simulink model "hug6dot_debug"  (R2021a)
settings: Solver=ode45  StartTime=0.0  StopTime=300  RelTol=1e-3
settings Model: Creator=daoist  LastModifiedBy=daoist

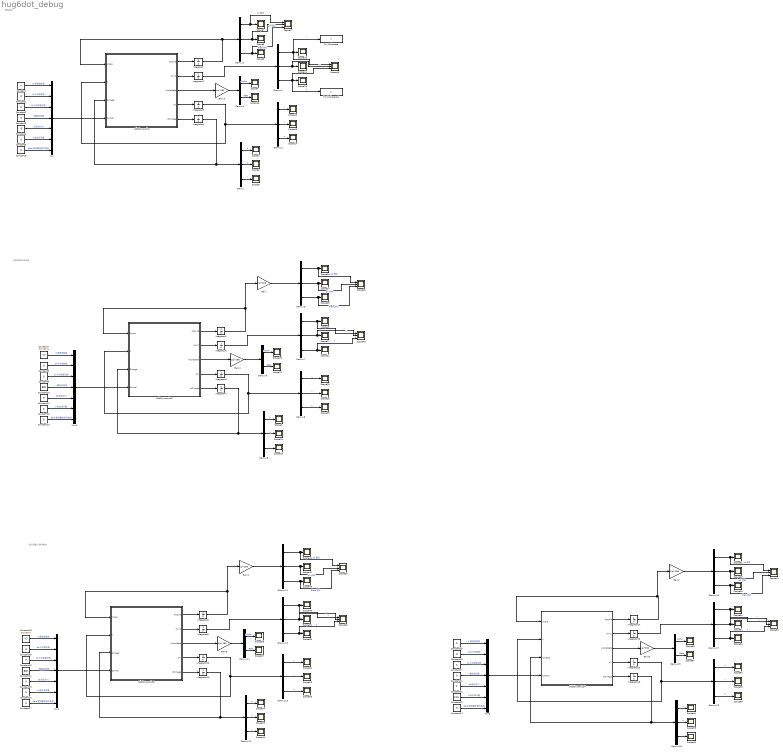
== system hug6dot_debug ==
  note: 验证忽略小项的影响
  note: 各种调试的实验场
  note: 原始版本
  6dotDynamics : Subsystem
  6dotDynamics2 : Subsystem
  6dotDynamics3 : Subsystem
  6dotDynamics4 : Subsystem
  Constant{,1..3,5..6,8..9,11..13,15..17,19..21,24..27} (21 alike) : Constant  Value=0
  Constant10 : Constant  Value=800
  Constant14 : Constant  Value=800
  Constant18 : Constant  Value=35/180*pi
  Constant22 : Constant  Value=2
  Constant23 : Constant  Value=0.01
  Constant4 : Constant  Value=-5
  Constant7 : Constant  Value=35/180*pi
  Demux{,1..3,5..8,10..13,15..18} (16 alike) : Demux  Outputs=3
  Demux{4,9,14,19} (4 alike) : Demux  Outputs=2
  Gain{,1..6} (7 alike) : Gain  Gain=1/pi*180
  Integrator{,1..2,4..5,7..9,11,13..15} (12 alike) : Integrator
  Integrator10 : Integrator  InitialCondition=[0.01 0 0]
  Integrator12 : Integrator  InitialCondition=[0.01 0 0]  UpperSaturationLimit=[inf 0.05 inf]  LowerSaturationLimit=-[inf 0.05 inf]
  Integrator3 : Integrator  InitialCondition=[0.01 0 0]
  Integrator6 : Integrator  InitialCondition=[0.01 0 0]
  Mux{,1..3} (4 alike) : Mux  Inputs=7
  Scope{1..28,31..43,45,51..64} (56 alike) : Scope
  Scope{29..30,44,46..50} (8 alike) : Scope  NumInputPorts=3
  To Workspace : ToWorkspace  VariableName=x  SampleTime=-1
  To Workspace1 : ToWorkspace  VariableName=z  SampleTime=-1
  wires:
  6dotDynamics/1(dAgnle) -> Integrator/1
  6dotDynamics/2(dXYZ) -> Integrator1/1
  6dotDynamics/4(dV) -> Integrator3/1
  6dotDynamics/5(dOmega) -> Integrator4/1
  Integrator4/1 -> 6dotDynamics/3(Omega), Demux/1
  Demux/1 -> Scope1/1  "p"
  Demux1/1 -> Scope47/1, Scope7/1  "psi横滚"
  Demux1/3 -> Scope47/3, Scope9/1  "theta俯仰"
  Integrator/1 -> Demux1/1, 6dotDynamics/1(Angle)
  Demux1/2 -> Scope47/2, Scope8/1  "phi回转"
  Demux3/1 -> Scope12/1  "u"
  Demux3/3 -> Scope14/1  "w"
  Integrator3/1 -> Demux3/1, 6dotDynamics/2(V)
  Demux3/2 -> Scope13/1  "v"
  Demux2/3 -> Scope46/3, To Workspace1/1, Scope15/1  "z"
  Demux2/1 -> Scope46/1, To Workspace/1, Scope10/1  "x"
  Demux2/2 -> Scope46/2, Scope11/1  "y"
  Integrator1/1 -> Demux2/1
  Demux/2 -> Scope5/1  "q"
  Demux/3 -> Scope6/1  "r"
  Demux4/1 -> Scope4/1  "Alpha"
  6dotDynamics/3(AlphaBeta) -> Gain3/1
  Demux4/2 -> Scope16/1  "Beta"
  Constant/1 -> Mux/1  "dr垂直舵舵角"
  Constant1/1 -> Mux/2  "de水平舵舵角"
  Constant2/1 -> Mux/3  "dd水平舵差动角"
  Constant3/1 -> Mux/4  "n螺旋桨转速"
  Constant4/1 -> Mux/5  "dB驱动浮力"
  Constant5/1 -> Mux/6  "dl姿态调节量"
  Constant6/1 -> Mux/7  "delta横滚重物调节角度"
  Mux/1 -> 6dotDynamics/4(Control)
  Mux1/1 -> 6dotDynamics2/4(Control)
  Constant13/1 -> Mux1/7  "delta横滚重物调节角度"
  Constant12/1 -> Mux1/6  "dl姿态调节量"
  Constant7/1 -> Mux1/1  "dr垂直舵舵角"
  Demux5/3 -> Scope25/1  "r"
  Demux5/2 -> Scope24/1  "q"
  Demux7/1 -> Scope49/1, Scope3/1  "x"
  6dotDynamics2/3(AlphaBeta) -> Gain4/1
  6dotDynamics2/5(dOmega) -> Integrator7/1
  Constant10/1 -> Mux1/4  "n螺旋桨转速"
  Demux7/2 -> Scope49/2, Scope17/1  "y"
  Demux9/1 -> Scope23/1  "Alpha"
  Demux7/3 -> Scope49/3, Scope21/1  "z"
  Demux9/2 -> Scope22/1  "Beta"
  Demux8/2 -> Scope19/1  "v"
  Demux6/1 -> Scope48/1, Scope26/1  "psi横滚"
  Demux6/3 -> Scope48/3, Scope28/1  "theta俯仰"
  Demux8/1 -> Scope18/1  "u"
  6dotDynamics2/1(dAgnle) -> Integrator2/1
  Demux5/1 -> Scope2/1  "p"
  Constant11/1 -> Mux1/5  "dB驱动浮力"
  Demux8/3 -> Scope20/1  "w"
  6dotDynamics2/4(dV) -> Integrator6/1
  Demux6/2 -> Scope48/2, Scope27/1  "phi回转"
  Integrator7/1 -> 6dotDynamics2/3(Omega), Demux5/1
  Constant9/1 -> Mux1/3  "dd水平舵差动角"
  Constant8/1 -> Mux1/2  "de水平舵舵角"
  Integrator6/1 -> Demux8/1, 6dotDynamics2/2(V)
  Integrator5/1 -> Demux7/1
  Integrator2/1 -> Gain/1, 6dotDynamics2/1(Angle)
  6dotDynamics2/2(dXYZ) -> Integrator5/1
  Gain/1 -> Demux6/1
  Constant16/1 -> Mux2/6  "dl姿态调节量"
  Constant19/1 -> Mux2/2  "de水平舵舵角"
  Constant20/1 -> Mux2/3  "dd水平舵差动角"
  Demux13/1 -> Scope32/1  "u"
  Integrator11/1 -> 6dotDynamics3/3(Omega), Demux10/1
  Demux11/2 -> Scope29/2, Scope42/1  "phi回转"
  6dotDynamics3/1(dAgnle) -> Integrator8/1
  Constant15/1 -> Mux2/5  "dB驱动浮力"
  Demux11/3 -> Scope29/3, Scope43/1  "theta俯仰"
  Demux10/2 -> Scope39/1  "q"
  Demux13/3 -> Scope35/1  "w"
  Integrator8/1 -> Gain1/1, 6dotDynamics3/1(Angle)
  Demux12/2 -> Scope30/2, Scope31/1  "y"
  Constant18/1 -> Mux2/1  "dr垂直舵舵角"
  Demux13/2 -> Scope33/1  "v"
  Mux2/1 -> 6dotDynamics3/4(Control)
  Integrator9/1 -> Demux12/1
  Demux14/1 -> Scope38/1  "Alpha"
  Integrator10/1 -> Demux13/1, 6dotDynamics3/2(V)
  Demux10/1 -> Scope34/1  "p"
  6dotDynamics3/3(AlphaBeta) -> Gain5/1
  Demux12/3 -> Scope30/3, Scope36/1  "z"
  Demux11/1 -> Scope29/1, Scope41/1  "psi横滚"
  6dotDynamics3/4(dV) -> Integrator10/1
  Demux12/1 -> Scope30/1, Scope45/1  "x"
  Demux14/2 -> Scope37/1  "Beta"
  Constant14/1 -> Mux2/4  "n螺旋桨转速"
  6dotDynamics3/2(dXYZ) -> Integrator9/1
  Gain1/1 -> Demux11/1
  Demux10/3 -> Scope40/1  "r"
  Constant17/1 -> Mux2/7  "delta横滚重物调节角度"
  6dotDynamics3/5(dOmega) -> Integrator11/1
  6dotDynamics4/5(dOmega) -> Integrator13/1
  Demux17/2 -> Scope50/2, Scope51/1  "y"
  Demux19/2 -> Scope57/1  "Beta"
  Mux3/1 -> 6dotDynamics4/4(Control)
  Gain2/1 -> Demux16/1
  Constant24/1 -> Mux3/7  "delta横滚重物调节角度"
  Integrator13/1 -> 6dotDynamics4/3(Omega), Demux15/1
  6dotDynamics4/3(AlphaBeta) -> Gain6/1
  Demux18/2 -> Scope53/1  "v"
  Demux17/1 -> Scope50/1, Scope64/1  "x"
  Demux15/2 -> Scope59/1  "q"
  Constant21/1 -> Mux3/4  "n螺旋桨转速"
  Integrator15/1 -> Demux17/1
  6dotDynamics4/2(dXYZ) -> Integrator15/1
  Demux19/1 -> Scope58/1  "Alpha"
  Demux15/3 -> Scope60/1  "r"
  Integrator14/1 -> Gain2/1, 6dotDynamics4/1(Angle)
  Constant26/1 -> Mux3/2  "de水平舵舵角"
  Constant25/1 -> Mux3/1  "dr垂直舵舵角"
  6dotDynamics4/4(dV) -> Integrator12/1
  Demux15/1 -> Scope54/1  "p"
  Demux16/1 -> Scope44/1, Scope61/1  "psi横滚"
  Integrator12/1 -> Demux18/1, 6dotDynamics4/2(V)
  Constant23/1 -> Mux3/6  "dl姿态调节量"
  6dotDynamics4/1(dAgnle) -> Integrator14/1
  Constant27/1 -> Mux3/3  "dd水平舵差动角"
  Demux18/1 -> Scope52/1  "u"
  Demux18/3 -> Scope55/1  "w"
  Demux16/3 -> Scope44/3, Scope63/1  "theta俯仰"
  Demux17/3 -> Scope50/3, Scope56/1  "z"
  Constant22/1 -> Mux3/5  "dB驱动浮力"
  Demux16/2 -> Scope44/2, Scope62/1  "phi回转"
  Gain3/1 -> Demux4/1
  Gain4/1 -> Demux9/1
  Gain5/1 -> Demux14/1
  Gain6/1 -> Demux19/1

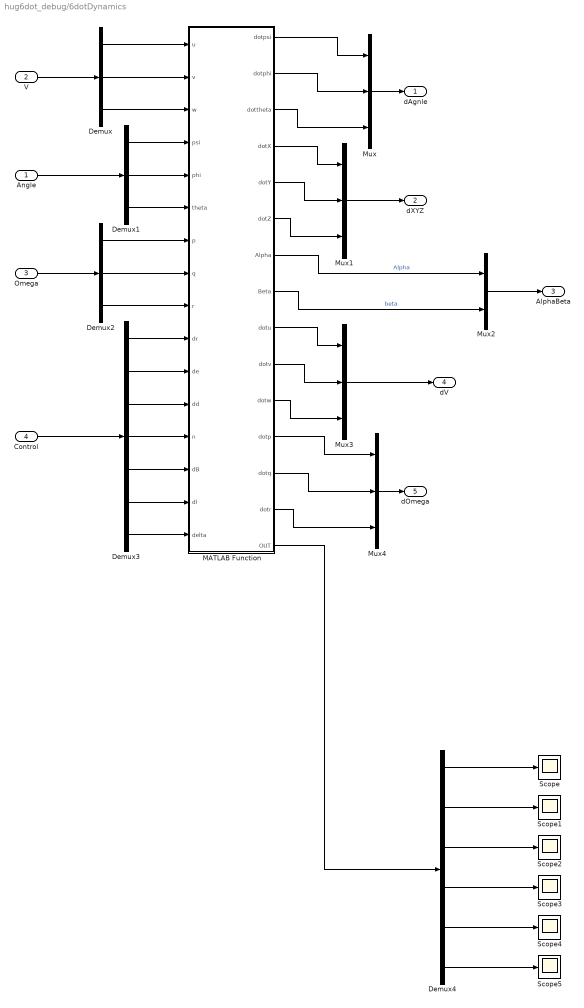
== system hug6dot_debug/6dotDynamics ==
  Angle : Inport
  V : Inport  Port=2
  Omega : Inport  Port=3
  Control : Inport  Port=4
  Demux : Demux  Outputs=3
  Demux1 : Demux  Outputs=3
  Demux2 : Demux  Outputs=3
  Demux3 : Demux  Outputs=7
  Demux4 : Demux  Outputs=6
  MATLAB Function : MATLAB Function  TreatAsAtomicUnit=on
  Mux{,1,3..4} (4 alike) : Mux  Inputs=3
  Mux2 : Mux  Inputs=2
  Scope{,1..5} (6 alike) : Scope
  dAgnle : Outport
  dXYZ : Outport  Port=2
  AlphaBeta : Outport  Port=3
  dV : Outport  Port=4
  dOmega : Outport  Port=5
  wires:
  MATLAB Function/6(dotZ) -> Mux1/3
  Mux1/1 -> dXYZ/1
  MATLAB Function/4(dotX) -> Mux1/1
  MATLAB Function/5(dotY) -> Mux1/2
  Mux/1 -> dAgnle/1
  MATLAB Function/7(Alpha) -> Mux2/1  "Alpha"
  MATLAB Function/8(Beta) -> Mux2/2  "beta"
  Mux2/1 -> AlphaBeta/1
  MATLAB Function/9(dotu) -> Mux3/1
  MATLAB Function/10(dotv) -> Mux3/2
  MATLAB Function/11(dotw) -> Mux3/3
  Mux3/1 -> dV/1
  MATLAB Function/12(dotp) -> Mux4/1
  MATLAB Function/13(dotq) -> Mux4/2
  MATLAB Function/14(dotr) -> Mux4/3
  Mux4/1 -> dOmega/1
  Demux/1 -> MATLAB Function/1(u)
  Demux/2 -> MATLAB Function/2(v)
  Demux/3 -> MATLAB Function/3(w)
  V/1 -> Demux/1
  Angle/1 -> Demux1/1
  Demux2/1 -> MATLAB Function/7(p)
  Demux2/2 -> MATLAB Function/8(q)
  Demux2/3 -> MATLAB Function/9(r)
  Omega/1 -> Demux2/1
  MATLAB Function/1(dotpsi) -> Mux/1
  MATLAB Function/2(dotphi) -> Mux/2
  MATLAB Function/3(dottheta) -> Mux/3
  Demux1/1 -> MATLAB Function/4(psi)
  Demux1/3 -> MATLAB Function/6(theta)
  Demux1/2 -> MATLAB Function/5(phi)
  Control/1 -> Demux3/1
  Demux3/1 -> MATLAB Function/10(dr)
  Demux3/2 -> MATLAB Function/11(de)
  Demux3/3 -> MATLAB Function/12(dd)
  Demux3/4 -> MATLAB Function/13(n)
  Demux3/5 -> MATLAB Function/14(dB)
  Demux3/6 -> MATLAB Function/15(dl)
  Demux3/7 -> MATLAB Function/16(delta)
  Demux4/1 -> Scope/1
  Demux4/5 -> Scope4/1
  Demux4/6 -> Scope5/1
  Demux4/4 -> Scope3/1
  Demux4/3 -> Scope2/1
  Demux4/2 -> Scope1/1
  MATLAB Function/15(OUT) -> Demux4/1

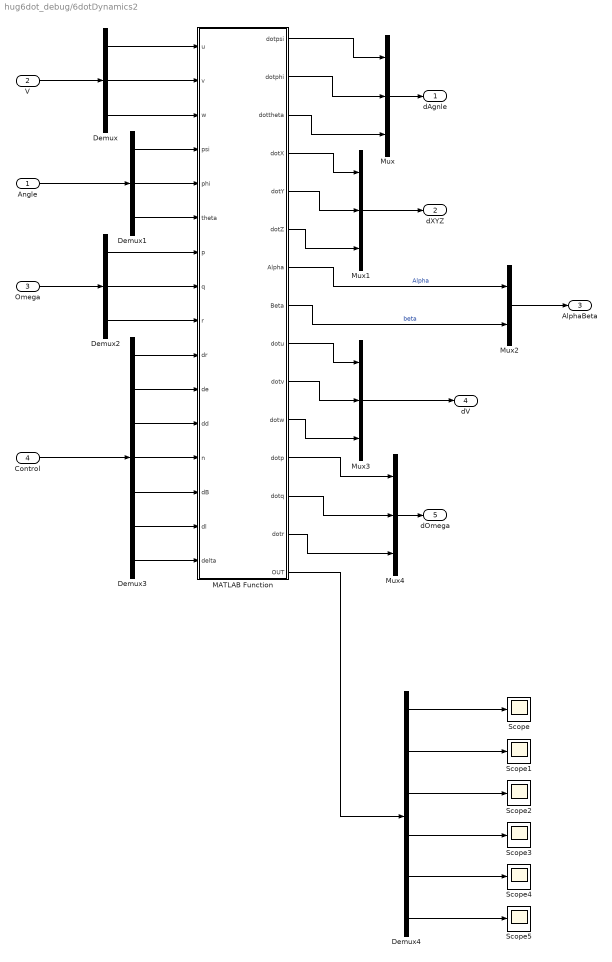
== system hug6dot_debug/6dotDynamics2 ==
  Angle : Inport
  V : Inport  Port=2
  Omega : Inport  Port=3
  Control : Inport  Port=4
  Demux : Demux  Outputs=3
  Demux1 : Demux  Outputs=3
  Demux2 : Demux  Outputs=3
  Demux3 : Demux  Outputs=7
  Demux4 : Demux  Outputs=6
  MATLAB Function : MATLAB Function  TreatAsAtomicUnit=on
  Mux{,1,3..4} (4 alike) : Mux  Inputs=3
  Mux2 : Mux  Inputs=2
  Scope{,1..5} (6 alike) : Scope
  dAgnle : Outport
  dXYZ : Outport  Port=2
  AlphaBeta : Outport  Port=3
  dV : Outport  Port=4
  dOmega : Outport  Port=5
  wires:
  MATLAB Function/6(dotZ) -> Mux1/3
  Mux1/1 -> dXYZ/1
  MATLAB Function/4(dotX) -> Mux1/1
  MATLAB Function/5(dotY) -> Mux1/2
  Mux/1 -> dAgnle/1
  MATLAB Function/7(Alpha) -> Mux2/1  "Alpha"
  MATLAB Function/8(Beta) -> Mux2/2  "beta"
  Mux2/1 -> AlphaBeta/1
  MATLAB Function/9(dotu) -> Mux3/1
  MATLAB Function/10(dotv) -> Mux3/2
  MATLAB Function/11(dotw) -> Mux3/3
  Mux3/1 -> dV/1
  MATLAB Function/12(dotp) -> Mux4/1
  MATLAB Function/13(dotq) -> Mux4/2
  MATLAB Function/14(dotr) -> Mux4/3
  Mux4/1 -> dOmega/1
  Demux/1 -> MATLAB Function/1(u)
  Demux/2 -> MATLAB Function/2(v)
  Demux/3 -> MATLAB Function/3(w)
  V/1 -> Demux/1
  Angle/1 -> Demux1/1
  Demux2/1 -> MATLAB Function/7(p)
  Demux2/2 -> MATLAB Function/8(q)
  Demux2/3 -> MATLAB Function/9(r)
  Omega/1 -> Demux2/1
  MATLAB Function/1(dotpsi) -> Mux/1
  MATLAB Function/2(dotphi) -> Mux/2
  MATLAB Function/3(dottheta) -> Mux/3
  Demux1/1 -> MATLAB Function/4(psi)
  Demux1/3 -> MATLAB Function/6(theta)
  Demux1/2 -> MATLAB Function/5(phi)
  Control/1 -> Demux3/1
  Demux3/1 -> MATLAB Function/10(dr)
  Demux3/2 -> MATLAB Function/11(de)
  Demux3/3 -> MATLAB Function/12(dd)
  Demux3/4 -> MATLAB Function/13(n)
  Demux3/5 -> MATLAB Function/14(dB)
  Demux3/6 -> MATLAB Function/15(dl)
  Demux3/7 -> MATLAB Function/16(delta)
  MATLAB Function/15(OUT) -> Demux4/1
  Demux4/1 -> Scope/1
  Demux4/2 -> Scope1/1
  Demux4/3 -> Scope2/1
  Demux4/4 -> Scope3/1
  Demux4/6 -> Scope5/1
  Demux4/5 -> Scope4/1

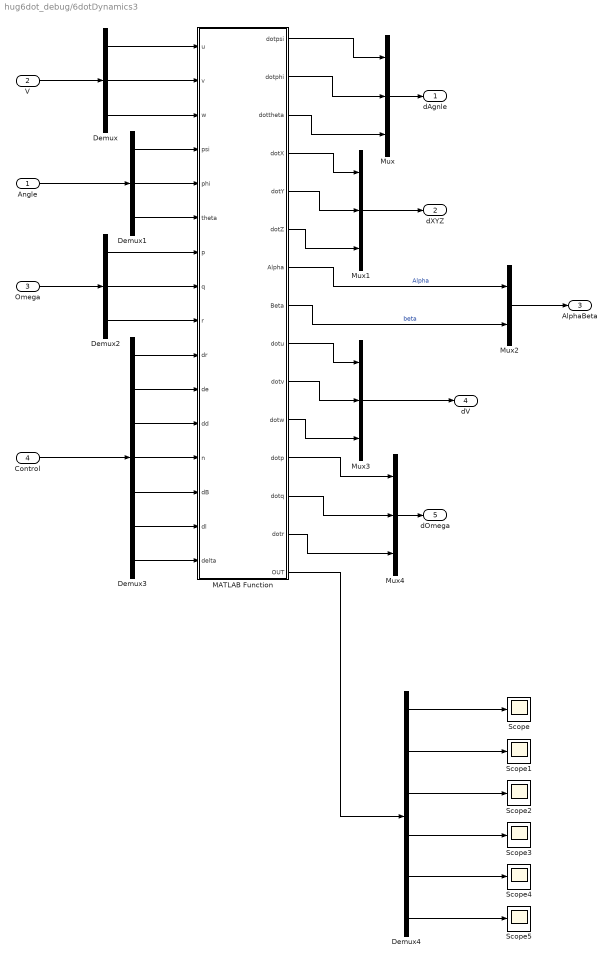
== system hug6dot_debug/6dotDynamics3 ==
  Angle : Inport
  V : Inport  Port=2
  Omega : Inport  Port=3
  Control : Inport  Port=4
  Demux : Demux  Outputs=3
  Demux1 : Demux  Outputs=3
  Demux2 : Demux  Outputs=3
  Demux3 : Demux  Outputs=7
  Demux4 : Demux  Outputs=6
  MATLAB Function : MATLAB Function  TreatAsAtomicUnit=on
  Mux{,1,3..4} (4 alike) : Mux  Inputs=3
  Mux2 : Mux  Inputs=2
  Scope{,1..5} (6 alike) : Scope
  dAgnle : Outport
  dXYZ : Outport  Port=2
  AlphaBeta : Outport  Port=3
  dV : Outport  Port=4
  dOmega : Outport  Port=5
  wires:
  MATLAB Function/6(dotZ) -> Mux1/3
  Mux1/1 -> dXYZ/1
  MATLAB Function/4(dotX) -> Mux1/1
  MATLAB Function/5(dotY) -> Mux1/2
  Mux/1 -> dAgnle/1
  MATLAB Function/7(Alpha) -> Mux2/1  "Alpha"
  MATLAB Function/8(Beta) -> Mux2/2  "beta"
  Mux2/1 -> AlphaBeta/1
  MATLAB Function/9(dotu) -> Mux3/1
  MATLAB Function/10(dotv) -> Mux3/2
  MATLAB Function/11(dotw) -> Mux3/3
  Mux3/1 -> dV/1
  MATLAB Function/12(dotp) -> Mux4/1
  MATLAB Function/13(dotq) -> Mux4/2
  MATLAB Function/14(dotr) -> Mux4/3
  Mux4/1 -> dOmega/1
  Demux/1 -> MATLAB Function/1(u)
  Demux/2 -> MATLAB Function/2(v)
  Demux/3 -> MATLAB Function/3(w)
  V/1 -> Demux/1
  Angle/1 -> Demux1/1
  Demux2/1 -> MATLAB Function/7(p)
  Demux2/2 -> MATLAB Function/8(q)
  Demux2/3 -> MATLAB Function/9(r)
  Omega/1 -> Demux2/1
  MATLAB Function/1(dotpsi) -> Mux/1
  MATLAB Function/2(dotphi) -> Mux/2
  MATLAB Function/3(dottheta) -> Mux/3
  Demux1/1 -> MATLAB Function/4(psi)
  Demux1/3 -> MATLAB Function/6(theta)
  Demux1/2 -> MATLAB Function/5(phi)
  Control/1 -> Demux3/1
  Demux3/1 -> MATLAB Function/10(dr)
  Demux3/2 -> MATLAB Function/11(de)
  Demux3/3 -> MATLAB Function/12(dd)
  Demux3/4 -> MATLAB Function/13(n)
  Demux3/5 -> MATLAB Function/14(dB)
  Demux3/6 -> MATLAB Function/15(dl)
  Demux3/7 -> MATLAB Function/16(delta)
  MATLAB Function/15(OUT) -> Demux4/1
  Demux4/1 -> Scope/1
  Demux4/2 -> Scope1/1
  Demux4/3 -> Scope2/1
  Demux4/4 -> Scope3/1
  Demux4/6 -> Scope5/1
  Demux4/5 -> Scope4/1

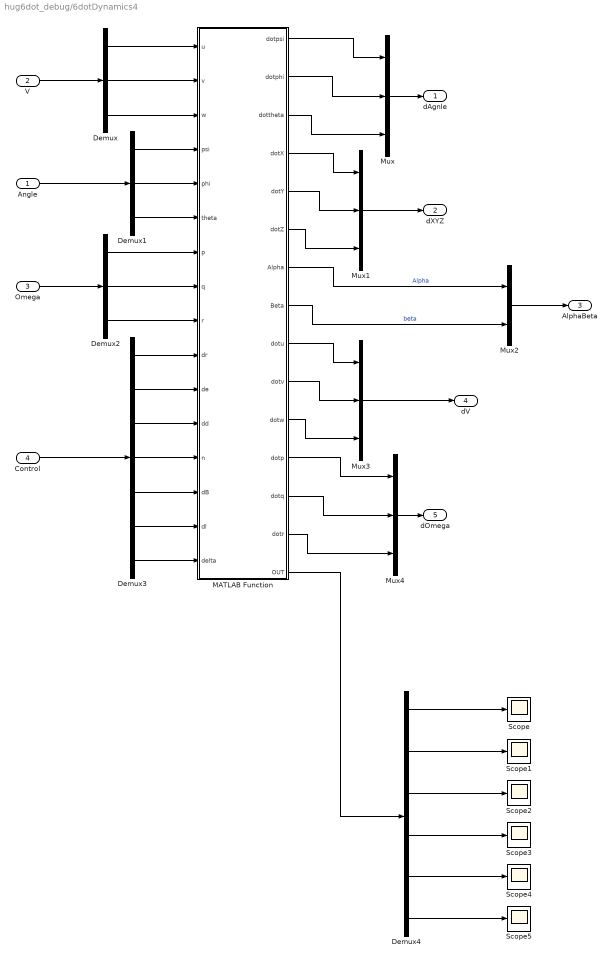
== system hug6dot_debug/6dotDynamics4 ==
  Angle : Inport
  V : Inport  Port=2
  Omega : Inport  Port=3
  Control : Inport  Port=4
  Demux : Demux  Outputs=3
  Demux1 : Demux  Outputs=3
  Demux2 : Demux  Outputs=3
  Demux3 : Demux  Outputs=7
  Demux4 : Demux  Outputs=6
  MATLAB Function : MATLAB Function  TreatAsAtomicUnit=on
  Mux{,1,3..4} (4 alike) : Mux  Inputs=3
  Mux2 : Mux  Inputs=2
  Scope{,1..5} (6 alike) : Scope
  dAgnle : Outport
  dXYZ : Outport  Port=2
  AlphaBeta : Outport  Port=3
  dV : Outport  Port=4
  dOmega : Outport  Port=5
  wires:
  MATLAB Function/6(dotZ) -> Mux1/3
  Mux1/1 -> dXYZ/1
  MATLAB Function/4(dotX) -> Mux1/1
  MATLAB Function/5(dotY) -> Mux1/2
  Mux/1 -> dAgnle/1
  MATLAB Function/7(Alpha) -> Mux2/1  "Alpha"
  MATLAB Function/8(Beta) -> Mux2/2  "beta"
  Mux2/1 -> AlphaBeta/1
  MATLAB Function/9(dotu) -> Mux3/1
  MATLAB Function/10(dotv) -> Mux3/2
  MATLAB Function/11(dotw) -> Mux3/3
  Mux3/1 -> dV/1
  MATLAB Function/12(dotp) -> Mux4/1
  MATLAB Function/13(dotq) -> Mux4/2
  MATLAB Function/14(dotr) -> Mux4/3
  Mux4/1 -> dOmega/1
  Demux/1 -> MATLAB Function/1(u)
  Demux/2 -> MATLAB Function/2(v)
  Demux/3 -> MATLAB Function/3(w)
  V/1 -> Demux/1
  Angle/1 -> Demux1/1
  Demux2/1 -> MATLAB Function/7(p)
  Demux2/2 -> MATLAB Function/8(q)
  Demux2/3 -> MATLAB Function/9(r)
  Omega/1 -> Demux2/1
  MATLAB Function/1(dotpsi) -> Mux/1
  MATLAB Function/2(dotphi) -> Mux/2
  MATLAB Function/3(dottheta) -> Mux/3
  Demux1/1 -> MATLAB Function/4(psi)
  Demux1/3 -> MATLAB Function/6(theta)
  Demux1/2 -> MATLAB Function/5(phi)
  Control/1 -> Demux3/1
  Demux3/1 -> MATLAB Function/10(dr)
  Demux3/2 -> MATLAB Function/11(de)
  Demux3/3 -> MATLAB Function/12(dd)
  Demux3/4 -> MATLAB Function/13(n)
  Demux3/5 -> MATLAB Function/14(dB)
  Demux3/6 -> MATLAB Function/15(dl)
  Demux3/7 -> MATLAB Function/16(delta)
  MATLAB Function/15(OUT) -> Demux4/1
  Demux4/1 -> Scope/1
  Demux4/2 -> Scope1/1
  Demux4/3 -> Scope2/1
  Demux4/4 -> Scope3/1
  Demux4/6 -> Scope5/1
  Demux4/5 -> Scope4/1

== matlab function hug6dot_debug/6dotDynamics3/MATLAB Function ==
  data: dotpsi output; u input; dotphi output; v input; w input; psi input; phi input; theta input; p input; q input; r input; dr input; de input; dd input; n input; dB input; dl input; dottheta output; dotX output; dotY output; dotZ output; Alpha output; Beta output; dotu output; dotv output; dotw output; dotp output; dotq output; dotr output; delta input; OUT output
function [ dotpsi,dotphi, dottheta, dotX, dotY, dotZ, Alpha, Beta, dotu,dotv,dotw,dotp,dotq,dotr, OUT] = Dynamics3(u,v,w,psi,phi,theta,p,q,r, dr,de,dd,n, dB,dl,delta)
% 混合驱动水下自航行器动力学行为与控制策略研究
rho = 1022;

m = 120;
G = 1176;
dG = 0;
S = 0.13;
xG = 0;
yG = -0.04;
zG = 0;
L = 3.2;

% 航行器对动坐标系的转动惯量
Jx = 2.45;
Jy = 87;
Jz = 87;

% 附加质量
lambda11 = 12;
lambda22 = 188.3;
lambda33 = 161;
% 附加静矩
% 问题：lambda26 应为负值，其余均为正值
lambda26 = -8.6;
lambda35 = 8.6;
% 附加惯矩
lambda44 = 0;
lambda55 = 110;
lambda66 = 110;

% 平移重物重力
Gm = 100;

% 螺旋桨推力系数
KT = 0.023;
% 螺旋桨直径
D = 0.25;

% 纵向力系数
% Cx = -0.16;
Cx0 = -0.16;
% 垂向力系数
Cay = 2.8;
Cry = 0.324;
Cdey = 1.01; %C_Y^{delta_e}
% 横向力系数
Cbz = -1.75;
Cpz = 0;
Cqz = -0.387;
Cdrz = -0.4;
% 横滚力矩系数
Cbr = 0;
Cpr = 0;
Cqr = 0;
Cdrr = 0;
Cddr = 0;
% 偏航力矩系数
Cbm = 0.47;
Cpm = 0;
Cqm = -0.14;
Cdrm = -0.47;
% 俯仰力矩系数
Can = 0.42;
Crn = -0.11;
Cden = -1.2;

% 横滚重物重力
Gr = 20;
% 横滚重物中心到转轴的距离
lr = 0.1;
% 螺旋桨力矩系数
Kq = 0.02;
% Kq = 0;



% Output = [dotu dotv dotw dotp dotq dotr]

% A = [m+lambda11,0,0, 0,0,0;
%     0, m+lambda22, 0,   0,0,m*xG+lambda26;
%     0,0,m+lambda33,0, -m*xG+lambda35,0;
%     0,0,0,Jx+lambda44,0,0;
%     0,0,-m*xG+lambda35,0,Jy+lambda55,0;
%     0,m*xG+lambda26,0,0,0,Jz+lambda66;];
% A = [m+lambda11,0,0, 0,m*zG,-m*yG;
%     0, m+lambda22, 0,   -m*zG,0,m*xG+lambda26;
%     0,0,m+lambda33, m*yG, -m*xG+lambda35,0;
%     0,-m*zG,m*yG,Jx+lambda44,0,0;
%     m*zG,0,-m*xG+lambda35,0,Jy+lambda55,0;
%     -m*yG,m*xG+lambda26,0,0,0,Jz+lambda66;];
% A = [m+lambda11,0,0, 0,0,-m*yG;
%     0, m+lambda22, 0,   0,0,lambda26;
%     0,0,m+lambda33, m*yG, lambda35,0;
%     0,0,m*yG,Jx+lambda44,0,0;
%     0,0,lambda35,0,Jy+lambda55,0;
%     -m*yG,lambda26,0,0,0,Jz+lambda66;];
% A = [m+lambda11,0,0, 0,0,0;
%     0, m+lambda22, 0,   0,0,lambda26;
%     0,0,m+lambda33, 0, lambda35,0;
%     0,0,0,Jx+lambda44,0,0;
%     0,0,lambda35,0,Jy+lambda55,0;
%     0,lambda26,0,0,0,Jz+lambda66;];

A = [m,0,0, 0,m*zG,-m*yG;
    0, m, 0,   -m*zG,0,m*xG;
    0,0,m, m*yG, -m*xG,0;
    0,-m*zG,m*yG,Jx,0,0;
    m*zG,0,-m*xG,0,Jy,0;
    -m*yG,m*xG,0,0,0,Jz;];

% A = [m,0,0, 0,0,0;
%     0, m, 0,   0,0,0;
%     0,0,m, 0, 0,0;
%     0,0,0,Jx,0,0;
%     0,0,0,0,Jy,0;
%     0,0,0,0,0,Jz;];

% 转换矩阵
% phi 航向角 绕y轴
% theta 俯仰角 绕z轴
% 横滚角 psi 绕x轴
RE1 = [cos(phi)  0 -sin(phi);
       0,1,0;
       sin(phi), 0, cos(phi);];
R12 = [cos(theta) sin(theta) 0;
    -sin(theta) cos(theta) 0;
    0,0,1;];
R2B = [1,0,0;
    0,cos(psi), sin(psi);
    0,-sin(psi), cos(psi);];
CEB = R2B * R12 * RE1;
CBE = CEB';
Cw = [1, -tan(theta)*cos(psi), tan(theta)*sin(psi);
    0, sin(psi), cos(psi);
    0, sec(theta)*cos(psi), -sec(theta)*sin(psi);];
Vt = sqrt(u^2 + v^2 + w^2);
Alpha = -atan(v/u);
Beta = asin(w/Vt);

p1 = p * L / Vt;
q1 = q * L / Vt;
r1 = r * L / Vt;

dotXYZ = CBE * [u v w]';
dotAngle = Cw * [p q r]';
dotX = dotXYZ(1);
dotY = dotXYZ(2);
dotZ = dotXYZ(3);
dotpsi = dotAngle(1);
dottheta = dotAngle(2);
dotphi = dotAngle(3);

 
 % 黏性类流体动力
% tau_v
Cy0 = 0;
Cz0 = 0;
mx0 = 0;
my0 = 0;
mz0 = 0;
Cx = Cx0 ;
Cy = Cy0 + Cay*Alpha + Cry*r1 + Cdey*de ;
Cz = Cz0 + Cbz*Beta + Cpz*p1 + Cqz*q1 + Cdrz*dr ;
mx = mx0 + Cbr*Beta + Cpr*p1 + Cqr*q1 + Cdrr*dr + Cddr*dd ;
my = my0 + Cbm*Beta + Cpm*p1 + Cqm*q1 + Cdrm*dr ;
mz = mz0 + Can*Alpha + Crn*r1 + Cden*de ;

Fxv = 0.5 * Cx * rho * Vt^2 * S;
Fyv = 0.5 * Cy * rho * Vt^2 * S;
Fzv = 0.5 * Cz * rho * Vt^2 * S;
Mxv = 0.5 * mx * rho * Vt^2 * S * L;
Myv = 0.5 * my * rho * Vt^2 * S * L;
Mzv = 0.5 * mz * rho * Vt^2 * S * L;

Fv = [Fxv, Fyv, Fzv]';
Mv = [Mxv, Myv, Mzv]';
Fv = zeros(3,1);
Mv = zeros(3,1);

% 负浮力A 
% G - B
FDG = CEB * [0, -dG, 0]';

% 姿态质量块

% 驱动浮力与驱动浮力矩
FDB = CEB * [0, -dB, 0]';
MB = cross([L/2,0,0]', FDB);

% 附加俯仰力矩及附加横滚力矩
FGm = CEB * [0,-Gm,0]';
MDM = cross([dl,0,0]', FGm);
Mr = [Gr*lr*sin(delta),0,0]';

% 推进器推力和转矩
T = [KT * rho * (D^4) * ((n/60)^2),0,0]';
MT = [-Kq * rho * (D^5) * ((n/60)^2),0,0]';

% 重力矩
FG = CEB * [0, -G, 0]';
RG = [xG,yG,zG]';
MG = cross(RG, FG);

% P1 = -m*(- v*r + w*q - xG*(q^2+r^2) + yG*p*q + zG*p*r);
% P2 = -m*(- w*q + u*r + xG*q*p - yG*(p^2+r^2) + zG*q*r);
% P3 = -m*(- u*q + v*p  + xG*r*p + yG*r*q - zG*(p^2+q^2));
% P4 = -((Jz-Jy)*q*r + m*(yG*(v*p-u*q) - zG*(u*r-w*q)));
% P5 = -((Jx-Jz)*r*p + m*(zG*(w*q-v*r) - xG*(v*p-u*q)));
% P6 = -((Jy-Jx)*p*q + m*(xG*(u*r-w*p) - yG*(w*q-v*r)));
P1 = -m*(- v*r);
P2 = -m*(  u*r );
P3 = -m*(- u*q );
P4 = -(  m*(yG*(-u*q) - zG*(u*r)));
P5 = -( - xG*(-u*q));
P6 = -(m*(xG*(u*r)));
P = [P1 P2 P3 P4 P5 P6]';
% P = zeros(6,1);

% CA * [V ;Omega]
out = inv(A) * ( P + [Fv+FDG+FDB+T;...
              Mv+MB+MDM+Mr+MT+MG;]);
OUT = ( P + [Fv+FDG+FDB+T;...
              Mv+MB+MDM+Mr+MT+MG;]);
dotu = out(1);
dotv = out(2);
dotw = out(3);
dotp = out(4);
dotq = out(5);
dotr = out(6);

== matlab function hug6dot_debug/6dotDynamics4/MATLAB Function ==
  data: dotpsi output; u input; dotphi output; v input; w input; psi input; phi input; theta input; p input; q input; r input; dr input; de input; dd input; n input; dB input; dl input; dottheta output; dotX output; dotY output; dotZ output; Alpha output; Beta output; dotu output; dotv output; dotw output; dotp output; dotq output; dotr output; delta input; OUT output
function [ dotpsi,dotphi, dottheta, dotX, dotY, dotZ, Alpha, Beta, dotu,dotv,dotw,dotp,dotq,dotr, OUT] = Dynamics4(u,v,w,psi,phi,theta,p,q,r, dr,de,dd,n, dB,dl,delta)
% 混合驱动水下自航行器动力学行为与控制策略研究
rho = 1022;

m = 69;
G = 676.2;
dG = 0;
S = 0.038;
xG = 0;
yG = -0.0047;
zG = 0;
L = 2.17;

% 航行器对动坐标系的转动惯量
Jx = 0;
Jy = 0;
Jz = 22.3;

% 附加质量
lambda11 = 2;
lambda22 = 75.8;
lambda33 = 0;
% 附加静矩
% 问题：lambda26 应为负值，其余均为正值
lambda26 = -12;
lambda35 = 0;
% 附加惯矩
lambda44 = 0;
lambda55 = 0;
lambda66 = 31;

% 平移重物重力
Gm = 180;

% 螺旋桨推力系数
KT = 0.34;
% 螺旋桨直径
D = 0.12;

% 纵向力系数
% Cx = -0.16;
Cx0 = -0.42;
% 垂向力系数
Cay = 0.316;
Cry = -8.37;
Cdey = 0; %C_Y^{delta_e}
% 横向力系数
Cbz = 0;
Cpz = 0;
Cqz = 0;
Cdrz = 0;
% 横滚力矩系数
Cbr = 0;
Cpr = 0;
Cqr = 0;
Cdrr = 0;
Cddr = 0;
% 偏航力矩系数
Cbm =0;
Cpm = 0;
Cqm = 0;
Cdrm = 0;
% 俯仰力矩系数
Can = -0.0573;
Crn = -2.34;
Cden = 0;

% 横滚重物重力
Gr = 0;
% 横滚重物中心到转轴的距离
lr = 0;
% 螺旋桨力矩系数
Kq = 0;

% Output = [dotu dotv dotw dotp dotq dotr]
AA = [m+lambda11,0,-m*yG;
    0, m+lambda22, m*xG+lambda26;
    -m*yG,m*xG+lambda26,Jz+lambda66;];
% A = [m+lambda11,0,0, 0,0,0;
%     0, m+lambda22, 0,   0,0,m*xG+lambda26;
%     0,0,m+lambda33,0, -m*xG+lambda35,0;
%     0,0,0,Jx+lambda44,0,0;
%     0,0,-m*xG+lambda35,0,Jy+lambda55,0;
%     0,m*xG+lambda26,0,0,0,Jz+lambda66;];
% A = [m+lambda11,0,0, 0,m*zG,-m*yG;
%     0, m+lambda22, 0,   -m*zG,0,m*xG+lambda26;
%     0,0,m+lambda33, m*yG, -m*xG+lambda35,0;
%     0,-m*zG,m*yG,Jx+lambda44,0,0;
%     m*zG,0,-m*xG+lambda35,0,Jy+lambda55,0;
%     -m*yG,m*xG+lambda26,0,0,0,Jz+lambda66;];
% A = [m+lambda11,0,0, 0,0,-m*yG;
%     0, m+lambda22, 0,   0,0,lambda26;
%     0,0,m+lambda33, m*yG, lambda35,0;
%     0,0,m*yG,Jx+lambda44,0,0;
%     0,0,lambda35,0,Jy+lambda55,0;
%     -m*yG,lambda26,0,0,0,Jz+lambda66;];
% A = [m+lambda11,0,0, 0,0,0;
%     0, m+lambda22, 0,   0,0,lambda26;
%     0,0,m+lambda33, 0, lambda35,0;
%     0,0,0,Jx+lambda44,0,0;
%     0,0,lambda35,0,Jy+lambda55,0;
%     0,lambda26,0,0,0,Jz+lambda66;];

% A = [m,0,0, 0,m*zG,-m*yG;
%     0, m, 0,   -m*zG,0,m*xG;
%     0,0,m, m*yG, -m*xG,0;
%     0,-m*zG,m*yG,Jx,0,0;
%     m*zG,0,-m*xG,0,Jy,0;
%     -m*yG,m*xG,0,0,0,Jz;];

% A = [m,0,0, 0,0,0;
%     0, m, 0,   0,0,0;
%     0,0,m, 0, 0,0;
%     0,0,0,Jx,0,0;
%     0,0,0,0,Jy,0;
%     0,0,0,0,0,Jz;];

% 转换矩阵
% phi 航向角 绕y轴
% theta 俯仰角 绕z轴
% 横滚角 psi 绕x轴
RE1 = [cos(phi)  0 -sin(phi);
       0,1,0;
       sin(phi), 0, cos(phi);];
R12 = [cos(theta) sin(theta) 0;
    -sin(theta) cos(theta) 0;
    0,0,1;];
R2B = [1,0,0;
    0,cos(psi), sin(psi);
    0,-sin(psi), cos(psi);];
CEB = R2B * R12 * RE1;
CBE = CEB';
Cw = [1, -tan(theta)*cos(psi), tan(theta)*sin(psi);
    0, sin(psi), cos(psi);
    0, sec(theta)*cos(psi), -sec(theta)*sin(psi);];
Vt = sqrt(u^2 + v^2 + w^2);
Alpha = -atan(v/u);
Beta = asin(w/Vt);

p1 = p * L / Vt;
q1 = q * L / Vt;
r1 = r * L / Vt;

dotXYZ = CBE * [u v w]';
dotAngle = Cw * [p q r]';
dotX = dotXYZ(1);
dotY = dotXYZ(2);
dotZ = dotXYZ(3);
dotpsi = dotAngle(1);
dottheta = dotAngle(2);
dotphi = dotAngle(3);

 
 % 黏性类流体动力
% tau_v
Cy0 = 0;
Cz0 = 0;
mx0 = 0;
my0 = 0;
mz0 = 0;
Cx = Cx0 ;
Cy = Cy0 + Cay*Alpha + Cry*r1 + Cdey*de ;
Cz = Cz0 + Cbz*Beta + Cpz*p1 + Cqz*q1 + Cdrz*dr ;
mx = mx0 + Cbr*Beta + Cpr*p1 + Cqr*q1 + Cdrr*dr + Cddr*dd ;
my = my0 + Cbm*Beta + Cpm*p1 + Cqm*q1 + Cdrm*dr ;
mz = mz0 + Can*Alpha + Crn*r1 + Cden*de ;

Fxv = 0.5 * Cx * rho * Vt^2 * S;
Fyv = 0.5 * Cy * rho * Vt^2 * S;
Fzv = 0.5 * Cz * rho * Vt^2 * S;
Mxv = 0.5 * mx * rho * Vt^2 * S * L;
Myv = 0.5 * my * rho * Vt^2 * S * L;
Mzv = 0.5 * mz * rho * Vt^2 * S * L;

Fv = [Fxv, Fyv, Fzv]';
Mv = [Mxv, Myv, Mzv]';
% Fv = zeros(3,1);
% Mv = zeros(3,1);

% 负浮力A 
% G - B
FDG = CEB * [0, -dG, 0]';

% 姿态质量块

% 驱动浮力与驱动浮力矩
lb = 0.93;
FDB = CEB * [0, -dB, 0]';
MB = cross([lb,0,0]', FDB);

% 附加俯仰力矩及附加横滚力矩
FGm = CEB * [0,-Gm,0]';
MDM = cross([dl,0,0]', FGm);
Mr = [Gr*lr*sin(delta),0,0]';

% 推进器推力和转矩
t = 0.16;
T = [KT * rho * (D^4) * ((n/60)^2),0,0]';
T = T * (1-t);
MT = [-Kq * rho * (D^5) * ((n/60)^2),0,0]';

% 重力矩
FG = CEB * [0, -G, 0]';
RG = [xG,yG,zG]';
MG = cross(RG, FG);

% P1 = -m*(- v*r + w*q - xG*(q^2+r^2) + yG*p*q + zG*p*r);
% P2 = -m*(- w*q + u*r + xG*q*p - yG*(p^2+r^2) + zG*q*r);
% P3 = -m*(- u*q + v*p  + xG*r*p + yG*r*q - zG*(p^2+q^2));
% P4 = -((Jz-Jy)*q*r + m*(yG*(v*p-u*q) - zG*(u*r-w*q)));
% P5 = -((Jx-Jz)*r*p + m*(zG*(w*q-v*r) - xG*(v*p-u*q)));
% P6 = -((Jy-Jx)*p*q + m*(xG*(u*r-w*p) - yG*(w*q-v*r)));
P1 = -m*(- v*r);
P2 = -m*(  u*r );
P3 = -m*(- u*q );
P4 = -(  m*(yG*(-u*q) - zG*(u*r)));
P5 = -( - xG*(-u*q));
P6 = -(m*(xG*(u*r)));
P = [P1 P2 P3 P4 P5 P6]';
% P = zeros(6,1);

% CA * [V ;Omega]
INVAA = inv(AA);
INVA = [INVAA(1,1) INVAA(1,2) 0 0 0 INVAA(1,3);
        INVAA(2,1) INVAA(2,2) 0 0 0 INVAA(2,3);
        zeros(6,1)';
        zeros(6,1)';
        zeros(6,1)';
        INVAA(3,1) INVAA(3,2) 0 0 0 INVAA(3,3);];
out = INVA * ( P + [Fv+FDG+FDB+T;...
              Mv+MB+MDM+Mr+MT+MG;]);
OUT = ( P + [Fv+FDG+FDB+T;...
              Mv+MB+MDM+Mr+MT+MG;]);
dotu = out(1);
dotv = out(2);
dotw = out(3);
dotp = out(4);
dotq = out(5);
dotr = out(6);

== matlab function hug6dot_debug/6dotDynamics2/MATLAB Function ==
  data: dotpsi output; u input; dotphi output; v input; w input; psi input; phi input; theta input; p input; q input; r input; dr input; de input; dd input; n input; dB input; dl input; dottheta output; dotX output; dotY output; dotZ output; Alpha output; Beta output; dotu output; dotv output; dotw output; dotp output; dotq output; dotr output; delta input; OUT output
function [ dotpsi,dotphi, dottheta, dotX, dotY, dotZ, Alpha, Beta, dotu,dotv,dotw,dotp,dotq,dotr, OUT] = Dynamics2(u,v,w,psi,phi,theta,p,q,r, dr,de,dd,n, dB,dl,delta)
% 混合驱动水下自航行器动力学行为与控制策略研究
rho = 1022;

m = 120;
G = 1176;
dG = 0;
S = 0.13;
xG = 0;
yG = -0.04;
zG = 0;
L = 3.2;

% 航行器对动坐标系的转动惯量
Jx = 2.45;
Jy = 87;
Jz = 87;

% 附加质量
lambda11 = 12;
lambda22 = 188.3;
lambda33 = 161;
% 附加静矩
% 问题：lambda26 应为负值，其余均为正值
lambda26 = -8.6;
lambda35 = 8.6;
% 附加惯矩
lambda44 = 0;
lambda55 = 110;
lambda66 = 110;

% 平移重物重力
Gm = 100;

% 螺旋桨推力系数
KT = 0.023;
% 螺旋桨直径
D = 0.25;

% 纵向力系数
% Cx = -0.16;
Cx0 = -0.16;
% 垂向力系数
Cay = 2.8;
Cry = 0.324;
Cdey = 1.01; %C_Y^{delta_e}
% 横向力系数
Cbz = -1.75;
Cpz = 0;
Cqz = -0.387;
Cdrz = -0.4;
% 横滚力矩系数
Cbr = 0;
Cpr = 0;
Cqr = 0;
Cdrr = 0;
Cddr = 0;
% 偏航力矩系数
Cbm = 0.47;
Cpm = 0;
Cqm = -0.14;
Cdrm = -0.47;
% 俯仰力矩系数
Can = 0.42;
Crn = -0.11;
Cden = -1.2;

% 横滚重物重力
Gr = 20;
% 横滚重物中心到转轴的距离
lr = 0.1;
% 螺旋桨力矩系数
Kq = 0.02;
% Kq = 0;



% Output = [dotu dotv dotw dotp dotq dotr]
% A = [m+lambda11,0,0, 0,m*zG,-m*yG;
%     0, m+lambda22, 0,   -m*zG,0,m*xG+lambda26;
%     0,0,m+lambda33, m*yG, -m*xG+lambda35,0;
%     0,-m*zG,m*yG,Jx+lambda44,0,0;
%     m*zG,0,-m*xG+lambda35,0,Jy+lambda55,0;
%     -m*yG,m*xG+lambda26,0,0,0,Jz+lambda66;];
% A = [m+lambda11,0,0, 0,0,-m*yG;
%     0, m+lambda22, 0,   0,0,lambda26;
%     0,0,m+lambda33, m*yG, lambda35,0;
%     0,0,m*yG,Jx+lambda44,0,0;
%     0,0,lambda35,0,Jy+lambda55,0;
%     -m*yG,lambda26,0,0,0,Jz+lambda66;];
% A = [m+lambda11,0,0, 0,0,0;
%     0, m+lambda22, 0,   0,0,lambda26;
%     0,0,m+lambda33, 0, lambda35,0;
%     0,0,0,Jx+lambda44,0,0;
%     0,0,lambda35,0,Jy+lambda55,0;
%     0,lambda26,0,0,0,Jz+lambda66;];

A = [m,0,0, 0,m*zG,-m*yG;
    0, m, 0,   -m*zG,0,m*xG;
    0,0,m, m*yG, -m*xG,0;
    0,-m*zG,m*yG,Jx,0,0;
    m*zG,0,-m*xG,0,Jy,0;
    -m*yG,m*xG,0,0,0,Jz;];

% A = [m,0,0, 0,0,0;
%     0, m, 0,   0,0,0;
%     0,0,m, 0, 0,0;
%     0,0,0,Jx,0,0;
%     0,0,0,0,Jy,0;
%     0,0,0,0,0,Jz;];
% A = [m+lambda11,0,0, 0,0,0;
%     0, m+lambda22, 0,   0,0,m*xG+lambda26;
%     0,0,m+lambda33, 0, -m*xG+lambda35,0;
%     0,0,0,Jx+lambda44,0,0;
%     0,0,-m*xG+lambda35,0,Jy+lambda55,0;
%     0,m*xG+lambda26,0,0,0,Jz+lambda66;];

% 转换矩阵
% phi 航向角 绕y轴
% theta 俯仰角 绕z轴
% 横滚角 psi 绕x轴
RE1 = [cos(phi)  0 -sin(phi);
       0,1,0;
       sin(phi), 0, cos(phi);];
R12 = [cos(theta) sin(theta) 0;
    -sin(theta) cos(theta) 0;
    0,0,1;];
R2B = [1,0,0;
    0,cos(psi), sin(psi);
    0,-sin(psi), cos(psi);];
CEB = R2B * R12 * RE1;
CBE = CEB';
% Cw = [1, -tan(theta)*cos(psi), tan(theta)*sin(psi);
%     0, sec(theta)*cos(psi), -sec(theta)*sin(psi);
%     0, sin(psi), cos(psi);];
Cw = [1, -tan(theta)*cos(psi), tan(theta)*sin(psi);
    0, sin(psi), cos(psi);
    0, sec(theta)*cos(psi), -sec(theta)*sin(psi);];
Vt = sqrt(u^2 + v^2 + w^2);
Alpha = -atan(v/u);
Beta = asin(w/Vt);

p1 = p * L / Vt;
q1 = q * L / Vt;
r1 = r * L / Vt;

dotXYZ = CBE * [u v w]';
dotAngle = Cw * [p q r]';
dotX = dotXYZ(1);
dotY = dotXYZ(2);
dotZ = dotXYZ(3);
dotpsi = dotAngle(1);
dottheta = dotAngle(2);
dotphi = dotAngle(3);

 
 % 黏性类流体动力
% tau_v
Cy0 = 0;
Cz0 = 0;
mx0 = 0;
my0 = 0;
mz0 = 0;
Cx = Cx0 ;
Cy = Cy0 + Cay*Alpha + Cry*r1 + Cdey*de ;
Cz = Cz0 + Cbz*Beta + Cpz*p1 + Cqz*q1 + Cdrz*dr ;
mx = mx0 + Cbr*Beta + Cpr*p1 + Cqr*q1 + Cdrr*dr + Cddr*dd ;
my = my0 + Cbm*Beta + Cpm*p1 + Cqm*q1 + Cdrm*dr ;
mz = mz0 + Can*Alpha + Crn*r1 + Cden*de ;

Fxv = 0.5 * Cx * rho * Vt^2 * S;
Fyv = 0.5 * Cy * rho * Vt^2 * S;
Fzv = 0.5 * Cz * rho * Vt^2 * S;
Mxv = 0.5 * mx * rho * Vt^2 * S * L;
Myv = 0.5 * my * rho * Vt^2 * S * L;
Mzv = 0.5 * mz * rho * Vt^2 * S * L;

Fv = [Fxv, Fyv, Fzv]';
Mv = [Mxv, Myv, Mzv]';
% Fv = zeros(3,1);
% Mv = zeros(3,1);

% 负浮力A 
% G - B
FDG = CEB * [0, -dG, 0]';

% 姿态质量块

% 驱动浮力与驱动浮力矩
FDB = CEB * [0, -dB, 0]';
MB = cross([L/2,0,0]', FDB);

% 附加俯仰力矩及附加横滚力矩
FGm = CEB * [0,-Gm,0]';
MDM = cross([dl,0,0]', FGm);
Mr = [Gr*lr*sin(delta),0,0]';

% 推进器推力和转矩
T = [KT * rho * (D^4) * ((n/60)^2),0,0]';
MT = [-Kq * rho * (D^5) * ((n/60)^2),0,0]';

% 重力矩
FG = CEB * [0, -G, 0]';
RG = [xG,yG,zG]';
MG = cross(RG, FG);

P1 = -m*(- v*r + w*q - xG*(q^2+r^2) + yG*p*q + zG*p*r);
P2 = -m*(- w*q + u*r + xG*q*p - yG*(p^2+r^2) + zG*q*r);
P3 = -m*(- u*q + v*p  + xG*r*p + yG*r*q - zG*(p^2+q^2));
P4 = -((Jz-Jy)*q*r + m*(yG*(v*p-u*q) - zG*(u*r-w*q)));
P5 = -((Jx-Jz)*r*p + m*(zG*(w*q-v*r) - xG*(v*p-u*q)));
P6 = -((Jy-Jx)*p*q + m*(xG*(u*r-w*p) - yG*(w*q-v*r)));

P = [P1 P2 P3 P4 P5 P6]';
% P = zeros(6,1);

% CA * [V ;Omega]
out = inv(A) * ( P + [Fv+FDG+FDB+T;...
              Mv+MB+MDM+Mr+MT+MG;]);
OUT = ( P + [Fv+FDG+FDB+T;...
              Mv+MB+MDM+Mr+MT+MG;]);
dotu = out(1);
dotv = out(2);
dotw = out(3);
dotp = out(4);
dotq = out(5);
dotr = out(6);

== matlab function hug6dot_debug/6dotDynamics/MATLAB Function ==
  data: dotpsi output; u input; dotphi output; v input; w input; psi input; phi input; theta input; p input; q input; r input; dr input; de input; dd input; n input; dB input; dl input; dottheta output; dotX output; dotY output; dotZ output; Alpha output; Beta output; dotu output; dotv output; dotw output; dotp output; dotq output; dotr output; delta input; OUT output
function [ dotpsi,dotphi, dottheta, dotX, dotY, dotZ, Alpha, Beta, dotu,dotv,dotw,dotp,dotq,dotr,OUT] = Dynamics(u,v,w,psi,phi,theta,p,q,r, dr,de,dd,n, dB,dl,delta)
% 混合驱动水下自航行器动力学行为与控制策略研究
rho = 1022;

m = 120;
G = 1176;
dG = 0;
S = 0.13;
xG = 0;
yG = -0.04;
zG = 0;
L = 3.2;

% 航行器对动坐标系的转动惯量
Jx = 2.45;
Jy = 87;
Jz = 87;

% 附加质量
lambda11 = 12;
lambda22 = 188.3;
lambda33 = 161;
% 附加静矩
lambda26 = -8.6;
lambda35 = 8.6;
% 附加惯矩
lambda44 = 0;
lambda55 = 110;
lambda66 = 110;

% 平移重物重力
Gm = 100;

% 螺旋桨推力系数
KT = 0.023;
% 螺旋桨直径
D = 0.25;

% 纵向力系数
Cx0 = -0.16;
% 垂向力系数
Cay = 2.8;
Cry = 0.324;
Cdey = 1.01; %C_Y^{delta_e}
% 横向力系数
Cbz = -1.75;
Cpz = 0;
Cqz = -0.387;
Cdrz = -0.4;
% 横滚力矩系数
Cbr = 0;
Cpr = 0;
Cqr = 0;
Cdrr = 0;
Cddr = 0;
% 偏航力矩系数
Cbm = 0.47;
Cpm = 0;
Cqm = -0.14;
Cdrm = -0.47;
% 俯仰力矩系数
Can = 0.42;
Crn = -0.11;
Cden = -1.2;

% 横滚重物重力
Gr = 20;
% 横滚重物中心到转轴的距离
lr = 0.1;
% 螺旋桨力矩系数
Kq = 0.02;
% Kq = 0;



% Output = [dotu dotv dotw dotp dotq dotr]
A = [m+lambda11,0,0, 0,m*zG,-m*yG;
    0, m+lambda22, 0,   -m*zG,0,m*xG+lambda26;
    0,0,m+lambda33, m*yG, -m*xG+lambda35,0;
    0,-m*zG,m*yG,Jx+lambda44,0,0;
    m*zG,0,-m*xG+lambda35,0,Jy+lambda55,0;
    -m*yG,m*xG+lambda26,0,0,0,Jz+lambda66;];


% 转换矩阵
% phi 航向角 绕y轴
% theta 俯仰角 绕z轴
% 横滚角 psi 绕x轴
RE1 = [cos(phi)  0 -sin(phi);
       0,1,0;
       sin(phi), 0, cos(phi);];
R12 = [cos(theta) sin(theta) 0;
       -sin(theta) cos(theta) 0;
       0,0,1;];
R2B = [1,0,0;
       0,cos(psi), sin(psi);
       0,-sin(psi), cos(psi);];
CEB = R2B * R12 * RE1;
CBE = CEB';
Cw = [1, -tan(theta)*cos(psi), tan(theta)*sin(psi);
      0, sec(theta)*cos(psi), -sec(theta)*sin(psi);
      0, sin(psi), cos(psi);];
Vt = sqrt(u^2 + v^2 + w^2);
Alpha = -atan(v/u);
Beta = asin(w/Vt);

p1 = p * L / Vt;
q1 = q * L / Vt;
r1 = r * L / Vt;

dotXYZ = CBE * [u v w]';
dotAngle = Cw * [p q r]';
dotX = dotXYZ(1);
dotY = dotXYZ(2);
dotZ = dotXYZ(3);
dotpsi = dotAngle(1);
dotphi = dotAngle(2);
dottheta = dotAngle(3);
 
 % 黏性类流体动力
% tau_v
Cy0 = 0;
Cz0 = 0;
mx0 = 0;
my0 = 0;
mz0 = 0;
Cx = Cx0 ;
Cy = Cy0 + Cay*Alpha + Cry*r1 + Cdey*de ;
Cz = Cz0 + Cbz*Beta + Cpz*p1 + Cqz*q1 + Cdrz*dr ;
mx = mx0 + Cbr*Beta + Cpr*p1 + Cqr*q1 + Cdrr*dr + Cddr*dd ;
my = my0 + Cbm*Beta + Cpm*p1 + Cqm*q1 + Cdrm*dr ;
mz = mz0 + Can*Alpha + Crn*r1 + Cden*de ;

Fxv = 0.5 * Cx * rho * Vt^2 * S;
Fyv = 0.5 * Cy * rho * Vt^2 * S;
Fzv = 0.5 * Cz * rho * Vt^2 * S;
Mxv = 0.5 * mx * rho * Vt^2 * S * L;
Myv = 0.5 * my * rho * Vt^2 * S * L;
Mzv = 0.5 * mz * rho * Vt^2 * S * L;
Fv = [Fxv, Fyv, Fzv]';
Mv = [Mxv, Myv, Mzv]';
% Fv = zeros(3,1);
% Mv = zeros(3,1);

% 负浮力A 
% G - B
FDG = CEB * [0, -dG, 0]';

% 驱动浮力与驱动浮力矩
FDB = CEB * [0, -dB, 0]';
MB = cross([L/2,0,0]', FDB);

% 附加俯仰力矩及附加横滚力矩
FGm = CEB * [0,-Gm,0]';
MDM = cross([dl,0,0]', FGm);
Mr = [Gr*lr*sin(delta),0,0]';

% 推进器推力和转矩
T = [KT * rho * (D^4) * ((n/60)^2),0,0]';
MT = [-Kq * rho * (D^5) * ((n/60)^2),0,0]';

% 重力矩
FG = CEB * [0, -G, 0]';
RG = [xG,yG,zG]';
MG = cross(RG, FG);

P1 = -m*(- v*r + w*q - xG*(q^2+r^2) + yG*p*q + zG*p*r);
P2 = -m*(- w*q + u*r + xG*q*p - yG*(p^2+r^2) + zG*q*r);
P3 = -m*(- u*q + v*p  + xG*r*p + yG*r*q - zG*(p^2+q^2));
P4 = -((Jz-Jy)*q*r + m*(yG*(v*p-u*q) - zG*(u*r-w*q)));
P5 = -((Jx-Jz)*r*p + m*(zG*(w*q-v*r) - xG*(v*p-w*q)));
P6 = -((Jy-Jx)*p*q + m*(xG*(u*r-w*p) - yG*(w*q-v*r)));

P = [P1 P2 P3 P4 P5 P6]';

% CA * [V ;Omega]
out = inv(A) * ( P + [Fv+FDG+FDB+T;...
              Mv+MB+MDM+Mr+MT+MG;]);
OUT = ([Fv+FDG+FDB+T;...
              Mv+MB+MDM+Mr+MT+MG;]);
dotu = out(1);
dotv = out(2);
dotw = out(3);
dotp = out(4);
dotq = out(5);
dotr = out(6);
